simulink model "generic_IVS"  (R2024a)
settings: Solver=FixedStepDiscrete  StartTime=0.0  StopTime=inf  FixedStep=0.001  RelTol=1e-3  EnableMultiTasking=on
undefined symbols (not defined in the file): carLengthObs, dir, ego_Accel, ego_Speed, ego_X, ego_Y, ego_YAW, goalPosTol, goalYawTol, init_CurrentLaneInfo, init_DrivingMissionInfo, init_EgoVehicle, init_HybridAStarParam, init_MapData, init_ParkingMIssionInfo, is_Optimal_Path, isPathFound, LAD, lane_Coeff, lane_Idx, lane_waypoints, lane_waypoints_Length, lookAheadDistance, maxIter, missionState, obsRadius, parking_clear, parkingDestinationPos_X, parkingDestinationPos_Y, parkingDestinationYaw, parkingMapBoundary_X_Max, parkingMapBoundary_X_Min, parkingMapBoundary_Y_Max, parkingMapBoundary_Y_Min, parkingStartPos_X, parkingStartPos_Y, R_min, reversePenalty, Route1, route1_waypoint, Route2, route2_waypoint, Route3, route3_waypoint, Route_Parking, route_parking_waypoint, steerSet, stepSize, tollgateLaneNumber, vehicleRadius, velReference, xyResolution, y_LAD, y_lookAheadDistance, yawResolution, yawWeight
libraries: CarMaker4SL x53, simulink x1
(part 3 of 4)

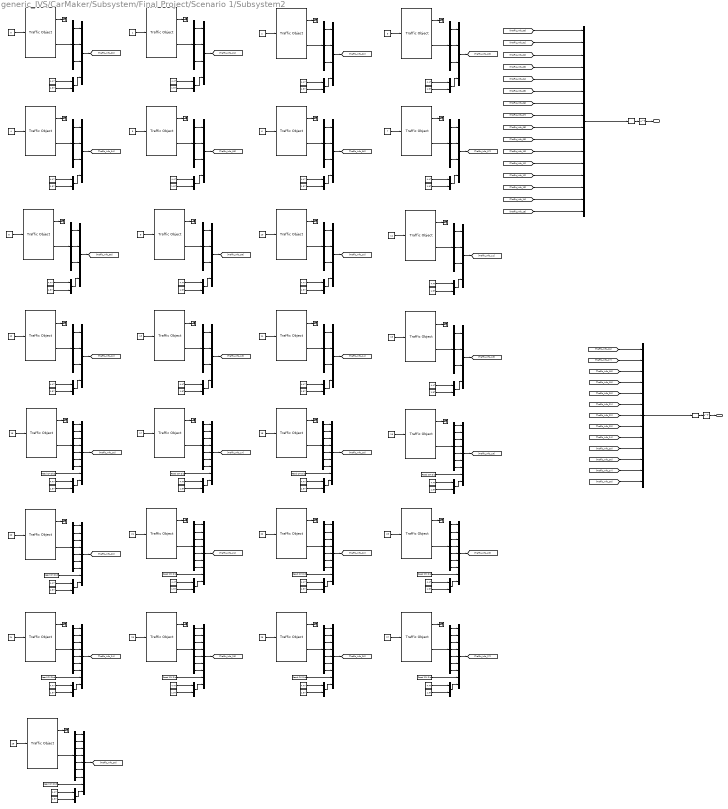
== system generic_IVS/CarMaker/Subsystem/Final Project/Scenario 1/Subsystem2 ==
  note: Traffic Size
      | Length: 4.47
      | Width: 1.97
      | Height: 1.12
  note: Traffic Size
      | Length: 4.47
      | Width: 1.97
      | Height: 1.12
  note: Traffic Size
      | Length: 4.47
      | Width: 1.97
      | Height: 1.12
  note: Traffic Size
      | Length: 4.47
      | Width: 1.97
      | Height: 1.12
  note: Traffic Size
      | Length: 4.47
      | Width: 1.97
      | Height: 1.12
  note: Traffic Size
      | Length: 4.47
      | Width: 1.97
      | Height: 1.12
  note: Traffic Size
      | Length: 4.47
      | Width: 1.97
      | Height: 1.12
  note: Traffic Size
      | Length: 4.47
      | Width: 1.97
      | Height: 1.12
  note: Traffic Size
      | Length: 4.47
      | Width: 1.97
      | Height: 1.12
  note: Traffic Size
      | Length: 4.47
      | Width: 1.97
      | Height: 1.12
  note: Traffic Size
      | Length: 4.47
      | Width: 1.97
      | Height: 1.12
  note: Traffic Size
      | Length: 4.47
      | Width: 1.97
      | Height: 1.12
  note: Traffic Size
      | Length: 4.47
      | Width: 1.97
      | Height: 1.12
  note: Traffic Size
      | Length: 4.47
      | Width: 1.97
      | Height: 1.12
  note: Traffic Size
      | Length: 4.47
      | Width: 1.97
      | Height: 1.12
  note: Traffic Size
      | Length: 4.47
      | Width: 1.97
      | Height: 1.12
  note: Traffic Size
      | Length: 4.47
      | Width: 1.97
      | Height: 1.12
  note: Traffic Size
      | Length: 4.47
      | Width: 1.97
      | Height: 1.12
  note: Traffic Size
      | Length: 4.47
      | Width: 1.97
      | Height: 1.12
  note: Traffic Size
      | Length: 4.47
      | Width: 1.97
      | Height: 1.12
  note: Traffic Size
      | Length: 4.47
      | Width: 1.97
      | Height: 1.12
  note: Traffic Size
      | Length: 4.47
      | Width: 1.97
      | Height: 1.12
  note: Traffic Size
      | Length: 4.47
      | Width: 1.97
      | Height: 1.12
  note: Traffic Size
      | Length: 4.47
      | Width: 1.97
      | Height: 1.12
  note: Traffic Size
      | Length: 4.47
      | Width: 1.97
      | Height: 1.12
  note: Traffic Size
      | Length: 4.47
      | Width: 1.97
      | Height: 1.12
  note: Traffic Size
      | Length: 4.47
      | Width: 1.97
      | Height: 1.12
  note: Traffic Size
      | Length: 4.47
      | Width: 1.97
      | Height: 1.12
  note: Traffic Size
      | Length: 4.47
      | Width: 1.97
      | Height: 1.12
  Bus Selector{1..14,19,29} (16 alike) : BusSelector  OutputSignals=t_0 x,t_0 y,r_zyx z
  Bus Selector{15..18,20..27,31} (13 alike) : BusSelector  OutputSignals=t_0 x,t_0 y,v_0 x,v_0 y,a_0 x,a_0 y,r_zyx z
  Constant1 : Constant
  Constant10 : Constant  Value=5
  Constant{2,5,8,11,14,17,19,23,26,29,31,35,38,41,43,47,50,53,55,59,62,65,67,71,74,77,79,89,94} (29 alike) : Constant  Value=4.47
  Constant{3,6,9,12,15,20..21,24,27,32..33,36,39,44..45,48,51,56..57,60,63,68..69,72,75,80..81,90,96} (29 alike) : Constant  Value=1.97
  Constant13 : Constant  Value=7
  Constant16 : Constant  Value=8
  Constant18 : Constant  Value=4
  Constant22 : Constant  Value=10
  Constant25 : Constant  Value=11
  Constant28 : Constant  Value=12
  Constant30 : Constant  Value=9
  Constant34 : Constant  Value=14
  Constant37 : Constant  Value=15
  Constant4 : Constant  Value=2
  Constant40 : Constant  Value=16
  Constant42 : Constant  Value=13
  Constant46 : Constant  Value=18
  Constant49 : Constant  Value=19
  Constant52 : Constant  Value=6
  Constant54 : Constant  Value=17
  Constant58 : Constant  Value=21
  Constant61 : Constant  Value=22
  Constant64 : Constant  Value=23
  Constant66 : Constant  Value=20
  Constant7 : Constant  Value=3
  Constant70 : Constant  Value=25
  Constant73 : Constant  Value=26
  Constant76 : Constant  Value=27
  Constant78 : Constant  Value=24
  Constant88 : Constant  Value=0
  Constant93 : Constant  Value=28
  Mux{1,3,5,7,10,12,14,16,18,20,22,24,26,30,36,60} (16 alike) : Mux
  Mux{2,4,6,8,11,13,15,17,19,21,23,25,27,29,31,33,35,37,39,41,43,45,47,49,51,53,55,61,65} (29 alike) : Mux  Inputs=2
  Mux{28,32,34,38,40,42,44,46,48,50,52,54,64} (13 alike) : Mux  Inputs=9
  Mux56 : Mux  Inputs=13
  Mux9 : Mux  Inputs=16
  Read CM Dict1 : CarMaker4SL/Read CM Dict  xname=Traffic.T20.rzv  xsync=off  xstime=Inherited
  Read CM Dict2 : CarMaker4SL/Read CM Dict  xname=Traffic.T18.rzv  xsync=off  xstime=Inherited
  Read CM Dict22 : CarMaker4SL/Read CM Dict  xname=Traffic.T21.rzv  xsync=off  xstime=Inherited
  Read CM Dict23 : CarMaker4SL/Read CM Dict  xname=Traffic.T22.rzv  xsync=off  xstime=Inherited
  Read CM Dict24 : CarMaker4SL/Read CM Dict  xname=Traffic.T23.rzv  xsync=off  xstime=Inherited
  Read CM Dict25 : CarMaker4SL/Read CM Dict  xname=Traffic.T24.rzv  xsync=off  xstime=Inherited
  Read CM Dict26 : CarMaker4SL/Read CM Dict  xname=Traffic.T25.rzv  xsync=off  xstime=Inherited
  Read CM Dict27 : CarMaker4SL/Read CM Dict  xname=Traffic.T26.rzv  xsync=off  xstime=Inherited
  Read CM Dict28 : CarMaker4SL/Read CM Dict  xname=Traffic.T27.rzv  xsync=off  xstime=Inherited
  Read CM Dict29 : CarMaker4SL/Read CM Dict  xname=Traffic.T28.rzv  xsync=off  xstime=Inherited
  Read CM Dict3 : CarMaker4SL/Read CM Dict  xname=Traffic.T17.rzv  xsync=off  xstime=Inherited
  Read CM Dict4 : CarMaker4SL/Read CM Dict  xname=Traffic.T16.rzv  xsync=off  xstime=Inherited
  Read CM Dict5 : CarMaker4SL/Read CM Dict  xname=Traffic.T19.rzv  xsync=off  xstime=Inherited
  Reshape : Reshape  OutputDimensionality=Customize  OutputDimensions=[5,16]
  Reshape1 : Reshape  OutputDimensionality=Customize  OutputDimensions=[10,13]
  Terminator{,1..28} (29 alike) : Terminator
  Traffic Object : CarMaker4SL/Traffic Object  xname=T00  ximode=Traffic Id  xstime=Inherited
      settings: SourceProductName=CarMaker4SL
  Traffic Object1 : CarMaker4SL/Traffic Object  xname=T01  ximode=Traffic Id  xstime=Inherited
      settings: SourceProductName=CarMaker4SL
  Traffic Object10 : CarMaker4SL/Traffic Object  xname=T11  ximode=Traffic Id  xstime=Inherited
      settings: SourceProductName=CarMaker4SL
  Traffic Object11 : CarMaker4SL/Traffic Object  xname=T12  ximode=Traffic Id  xstime=Inherited
      settings: SourceProductName=CarMaker4SL
  Traffic Object12 : CarMaker4SL/Traffic Object  xname=T13  ximode=Traffic Id  xstime=Inherited
      settings: SourceProductName=CarMaker4SL
  Traffic Object13 : CarMaker4SL/Traffic Object  xname=T14  ximode=Traffic Id  xstime=Inherited
      settings: SourceProductName=CarMaker4SL
  Traffic Object14 : CarMaker4SL/Traffic Object  xname=T15  ximode=Traffic Id  xstime=Inherited
      settings: SourceProductName=CarMaker4SL
  Traffic Object15 : CarMaker4SL/Traffic Object  xname=T16  ximode=Traffic Id  xstime=Inherited
      settings: SourceProductName=CarMaker4SL
  Traffic Object16 : CarMaker4SL/Traffic Object  xname=T17  ximode=Traffic Id  xstime=Inherited
      settings: SourceProductName=CarMaker4SL
  Traffic Object17 : CarMaker4SL/Traffic Object  xname=T18  ximode=Traffic Id  xstime=Inherited
      settings: SourceProductName=CarMaker4SL
  Traffic Object18 : CarMaker4SL/Traffic Object  xname=T19  ximode=Traffic Id  xstime=Inherited
      settings: SourceProductName=CarMaker4SL
  Traffic Object19 : CarMaker4SL/Traffic Object  xname=T06  ximode=Traffic Id  xstime=Inherited
      settings: SourceProductName=CarMaker4SL
  Traffic Object2 : CarMaker4SL/Traffic Object  xname=T02  ximode=Traffic Id  xstime=Inherited
      settings: SourceProductName=CarMaker4SL
  Traffic Object20 : CarMaker4SL/Traffic Object  xname=T20  ximode=Traffic Id  xstime=Inherited
      settings: SourceProductName=CarMaker4SL
  Traffic Object21 : CarMaker4SL/Traffic Object  xname=T21  ximode=Traffic Id  xstime=Inherited
      settings: SourceProductName=CarMaker4SL
  Traffic Object22 : CarMaker4SL/Traffic Object  xname=T22  ximode=Traffic Id  xstime=Inherited
      settings: SourceProductName=CarMaker4SL
  Traffic Object23 : CarMaker4SL/Traffic Object  xname=T23  ximode=Traffic Id  xstime=Inherited
      settings: SourceProductName=CarMaker4SL
  Traffic Object24 : CarMaker4SL/Traffic Object  xname=T24  ximode=Traffic Id  xstime=Inherited
      settings: SourceProductName=CarMaker4SL
  Traffic Object25 : CarMaker4SL/Traffic Object  xname=T25  ximode=Traffic Id  xstime=Inherited
      settings: SourceProductName=CarMaker4SL
  Traffic Object26 : CarMaker4SL/Traffic Object  xname=T26  ximode=Traffic Id  xstime=Inherited
      settings: SourceProductName=CarMaker4SL
  Traffic Object27 : CarMaker4SL/Traffic Object  xname=T27  ximode=Traffic Id  xstime=Inherited
      settings: SourceProductName=CarMaker4SL
  Traffic Object28 : CarMaker4SL/Traffic Object  xname=T28  ximode=Traffic Id  xstime=Inherited
      settings: SourceProductName=CarMaker4SL
  Traffic Object3 : CarMaker4SL/Traffic Object  xname=T03  ximode=Traffic Id  xstime=Inherited
      settings: SourceProductName=CarMaker4SL
  Traffic Object4 : CarMaker4SL/Traffic Object  xname=T04  ximode=Traffic Id  xstime=Inherited
      settings: SourceProductName=CarMaker4SL
  Traffic Object5 : CarMaker4SL/Traffic Object  xname=T05  ximode=Traffic Id  xstime=Inherited
      settings: SourceProductName=CarMaker4SL
  Traffic Object6 : CarMaker4SL/Traffic Object  xname=T07  ximode=Traffic Id  xstime=Inherited
      settings: SourceProductName=CarMaker4SL
  Traffic Object7 : CarMaker4SL/Traffic Object  xname=T08  ximode=Traffic Id  xstime=Inherited
      settings: SourceProductName=CarMaker4SL
  Traffic Object8 : CarMaker4SL/Traffic Object  xname=T09  ximode=Traffic Id  xstime=Inherited
      settings: SourceProductName=CarMaker4SL
  Traffic Object9 : CarMaker4SL/Traffic Object  xname=T10  ximode=Traffic Id  xstime=Inherited
      settings: SourceProductName=CarMaker4SL
  Transpose : Math  Operator=transpose
  Transpose1 : Math  Operator=transpose
  Traffic_Parking : Outport
  Traaffic_Info : Outport  Port=2
  wires:
  [Traffic_Info_00] -> Mux9/1
  [Traffic_Info_01] -> Mux9/2
  [Traffic_Info_02] -> Mux9/3
  [Traffic_Info_06] -> Mux9/7
  [Traffic_Info_05] -> Mux9/6
  [Traffic_Info_04] -> Mux9/5
  [Traffic_Info_03] -> Mux9/4
  [Traffic_Info_09] -> Mux9/10
  [Traffic_Info_10] -> Mux9/11
  [Traffic_Info_11] -> Mux9/12
  [Traffic_Info_08] -> Mux9/9
  [Traffic_Info_12] -> Mux9/13
  [Traffic_Info_13] -> Mux9/14
  [Traffic_Info_07] -> Mux9/8
  [Traffic_Info_15] -> Mux9/16
  [Traffic_Info_14] -> Mux9/15
  Traffic Object/2 -> Bus Selector29/1
  Constant88/1 -> Traffic Object/1
  Traffic Object/1 -> Terminator/1
  Bus Selector29/1 -> Mux60/1  "<t_0 x>"
  Bus Selector29/2 -> Mux60/2  "<t_0 y>"
  Bus Selector29/3 -> Mux60/3  "<r_zyx z>"
  Mux60/1 -> [Traffic_Info_00]
  Constant89/1 -> Mux61/1
  Constant90/1 -> Mux61/2
  Mux61/1 -> Mux60/4
  Bus Selector23/5 -> Mux44/5  "<a_0 x>"
  Traffic Object22/2 -> Bus Selector21/1
  Mux41/1 -> Mux40/9
  Constant63/1 -> Mux43/2
  Bus Selector23/2 -> Mux44/2  "<t_0 y>"
  Bus Selector21/2 -> Mux42/2  "<t_0 y>"
  Bus Selector21/5 -> Mux42/5  "<a_0 x>"
  Traffic Object22/1 -> Terminator22/1
  Bus Selector23/6 -> Mux44/6  "<a_0 y>"
  Bus Selector23/7 -> Mux44/7  "<r_zyx z>"
  Traffic Object23/1 -> Terminator23/1
  Traffic Object23/2 -> Bus Selector23/1
  Constant68/1 -> Mux45/2
  Mux45/1 -> Mux44/9
  Constant61/1 -> Traffic Object22/1
  Read CM Dict24/1 -> Mux44/8
  Mux42/1 -> [Traffic_Info_22]
  Mux40/1 -> [Traffic_Info_21]
  Mux44/1 -> [Traffic_Info_23]
  Bus Selector23/4 -> Mux44/4  "<v_0 y>"
  Bus Selector21/6 -> Mux42/6  "<a_0 y>"
  Bus Selector20/6 -> Mux40/6  "<a_0 y>"
  Bus Selector21/3 -> Mux42/3  "<v_0 x>"
  Bus Selector21/4 -> Mux42/4  "<v_0 y>"
  Bus Selector21/1 -> Mux42/1  "<t_0 x>"
  Constant58/1 -> Traffic Object21/1
  Bus Selector21/7 -> Mux42/7  "<r_zyx z>"
  Constant65/1 -> Mux45/1
  Bus Selector20/1 -> Mux40/1  "<t_0 x>"
  Bus Selector23/1 -> Mux44/1  "<t_0 x>"
  Bus Selector20/3 -> Mux40/3  "<v_0 x>"
  Constant60/1 -> Mux41/2
  Traffic Object21/2 -> Bus Selector20/1
  Read CM Dict22/1 -> Mux40/8
  Bus Selector20/5 -> Mux40/5  "<a_0 x>"
  Traffic Object21/1 -> Terminator21/1
  Bus Selector20/2 -> Mux40/2  "<t_0 y>"
  Bus Selector23/3 -> Mux44/3  "<v_0 x>"
  Constant64/1 -> Traffic Object23/1
  Bus Selector20/7 -> Mux40/7  "<r_zyx z>"
  Read CM Dict23/1 -> Mux42/8
  Constant62/1 -> Mux43/1
  Bus Selector20/4 -> Mux40/4  "<v_0 y>"
  Constant59/1 -> Mux41/1
  Mux43/1 -> Mux42/9
  Bus Selector26/3 -> Mux54/3  "<v_0 x>"
  Bus Selector27/5 -> Mux52/5  "<a_0 x>"
  Bus Selector26/5 -> Mux54/5  "<a_0 x>"
  Traffic Object26/2 -> Bus Selector25/1
  Bus Selector26/6 -> Mux54/6  "<a_0 y>"
  Mux49/1 -> Mux48/9
  Constant75/1 -> Mux51/2
  Bus Selector27/2 -> Mux52/2  "<t_0 y>"
  Bus Selector25/2 -> Mux50/2  "<t_0 y>"
  Bus Selector25/5 -> Mux50/5  "<a_0 x>"
  Traffic Object26/1 -> Terminator26/1
  Bus Selector27/6 -> Mux52/6  "<a_0 y>"
  Bus Selector26/7 -> Mux54/7  "<r_zyx z>"
  Bus Selector27/7 -> Mux52/7  "<r_zyx z>"
  Bus Selector26/1 -> Mux54/1  "<t_0 x>"
  Traffic Object27/1 -> Terminator27/1
  Traffic Object27/2 -> Bus Selector27/1
  Constant80/1 -> Mux53/2
  Mux53/1 -> Mux52/9
  Constant73/1 -> Traffic Object26/1
  Read CM Dict28/1 -> Mux52/8
  Mux50/1 -> [Traffic_Info_26]
  Mux48/1 -> [Traffic_Info_25]
  Mux52/1 -> [Traffic_Info_27]
  Bus Selector27/4 -> Mux52/4  "<v_0 y>"
  Constant78/1 -> Traffic Object24/1
  Traffic Object24/1 -> Terminator24/1
  Bus Selector25/6 -> Mux50/6  "<a_0 y>"
  Bus Selector24/6 -> Mux48/6  "<a_0 y>"
  Bus Selector25/3 -> Mux50/3  "<v_0 x>"
  Read CM Dict25/1 -> Mux54/8
  Bus Selector25/4 -> Mux50/4  "<v_0 y>"
  Bus Selector26/4 -> Mux54/4  "<v_0 y>"
  Bus Selector25/1 -> Mux50/1  "<t_0 x>"
  Constant70/1 -> Traffic Object25/1
  Bus Selector25/7 -> Mux50/7  "<r_zyx z>"
  Constant77/1 -> Mux53/1
  Bus Selector26/2 -> Mux54/2  "<t_0 y>"
  Bus Selector24/1 -> Mux48/1  "<t_0 x>"
  Bus Selector27/1 -> Mux52/1  "<t_0 x>"
  Bus Selector24/3 -> Mux48/3  "<v_0 x>"
  Mux54/1 -> [Traffic_Info_24]
  Constant72/1 -> Mux49/2
  Traffic Object25/2 -> Bus Selector24/1
  Read CM Dict26/1 -> Mux48/8
  Bus Selector24/5 -> Mux48/5  "<a_0 x>"
  Traffic Object25/1 -> Terminator25/1
  Constant81/1 -> Mux55/2
  Bus Selector24/2 -> Mux48/2  "<t_0 y>"
  Bus Selector27/3 -> Mux52/3  "<v_0 x>"
  Constant76/1 -> Traffic Object27/1
  Bus Selector24/7 -> Mux48/7  "<r_zyx z>"
  Traffic Object24/2 -> Bus Selector26/1
  Read CM Dict27/1 -> Mux50/8
  Mux55/1 -> Mux54/9
  Constant74/1 -> Mux51/1
  Bus Selector24/4 -> Mux48/4  "<v_0 y>"
  Constant71/1 -> Mux49/1
  Constant79/1 -> Mux55/1
  Mux51/1 -> Mux50/9
  Bus Selector31/3 -> Mux64/3  "<v_0 x>"
  Bus Selector31/5 -> Mux64/5  "<a_0 x>"
  Bus Selector31/6 -> Mux64/6  "<a_0 y>"
  Bus Selector31/7 -> Mux64/7  "<r_zyx z>"
  Bus Selector31/1 -> Mux64/1  "<t_0 x>"
  Constant93/1 -> Traffic Object28/1
  Traffic Object28/1 -> Terminator28/1
  Read CM Dict29/1 -> Mux64/8
  Bus Selector31/4 -> Mux64/4  "<v_0 y>"
  Bus Selector31/2 -> Mux64/2  "<t_0 y>"
  Mux64/1 -> [Traffic_Info_28]
  Constant96/1 -> Mux65/2
  Traffic Object28/2 -> Bus Selector31/1
  Mux65/1 -> Mux64/9
  Constant94/1 -> Mux65/1
  Bus Selector1/3 -> Mux1/3  "<r_zyx z>"
  Mux1/1 -> [Traffic_Info_01]
  Bus Selector1/1 -> Mux1/1  "<t_0 x>"
  Traffic Object1/1 -> Terminator1/1
  Constant2/1 -> Mux2/1
  Constant3/1 -> Mux2/2
  Bus Selector1/2 -> Mux1/2  "<t_0 y>"
  Mux2/1 -> Mux1/4
  Constant1/1 -> Traffic Object1/1
  Traffic Object1/2 -> Bus Selector1/1
  Bus Selector2/3 -> Mux3/3  "<r_zyx z>"
  Mux3/1 -> [Traffic_Info_02]
  Bus Selector2/1 -> Mux3/1  "<t_0 x>"
  Traffic Object2/1 -> Terminator2/1
  Constant5/1 -> Mux4/1
  Constant6/1 -> Mux4/2
  Bus Selector2/2 -> Mux3/2  "<t_0 y>"
  Mux4/1 -> Mux3/4
  Constant4/1 -> Traffic Object2/1
  Traffic Object2/2 -> Bus Selector2/1
  Bus Selector3/3 -> Mux5/3  "<r_zyx z>"
  Mux5/1 -> [Traffic_Info_03]
  Bus Selector3/1 -> Mux5/1  "<t_0 x>"
  Traffic Object3/1 -> Terminator3/1
  Constant8/1 -> Mux6/1
  Constant9/1 -> Mux6/2
  Bus Selector3/2 -> Mux5/2  "<t_0 y>"
  Mux6/1 -> Mux5/4
  Constant7/1 -> Traffic Object3/1
  Traffic Object3/2 -> Bus Selector3/1
  Bus Selector6/3 -> Mux14/3  "<r_zyx z>"
  Mux14/1 -> [Traffic_Info_04]
  Bus Selector6/1 -> Mux14/1  "<t_0 x>"
  Mux8/1 -> Mux7/4
  Constant12/1 -> Mux8/2
  Mux7/1 -> [Traffic_Info_05]
  Traffic Object4/1 -> Terminator4/1
  Bus Selector4/2 -> Mux7/2  "<t_0 y>"
  Constant18/1 -> Traffic Object4/1
  Constant21/1 -> Mux15/2
  Constant10/1 -> Traffic Object5/1
  Bus Selector6/2 -> Mux14/2  "<t_0 y>"
  Mux15/1 -> Mux14/4
  Traffic Object4/2 -> Bus Selector6/1
  Constant16/1 -> Traffic Object7/1
  Traffic Object7/2 -> Bus Selector7/1
  Constant17/1 -> Mux13/1
  Constant19/1 -> Mux15/1
  Constant11/1 -> Mux8/1
  Traffic Object7/1 -> Terminator7/1
  Constant20/1 -> Mux13/2
  Bus Selector4/1 -> Mux7/1  "<t_0 x>"
  Mux13/1 -> Mux12/4
  Bus Selector7/1 -> Mux12/1  "<t_0 x>"
  Bus Selector4/3 -> Mux7/3  "<r_zyx z>"
  Bus Selector7/3 -> Mux12/3  "<r_zyx z>"
  Mux12/1 -> [Traffic_Info_08]
  Constant15/1 -> Mux11/2
  Mux11/1 -> Mux10/4
  Constant13/1 -> Traffic Object6/1
  Traffic Object5/1 -> Terminator5/1
  Constant14/1 -> Mux11/1
  Traffic Object6/1 -> Terminator6/1
  Traffic Object5/2 -> Bus Selector4/1
  Bus Selector5/1 -> Mux10/1  "<t_0 x>"
  Bus Selector7/2 -> Mux12/2  "<t_0 y>"
  Traffic Object6/2 -> Bus Selector5/1
  Bus Selector5/3 -> Mux10/3  "<r_zyx z>"
  Mux10/1 -> [Traffic_Info_07]
  Bus Selector5/2 -> Mux10/2  "<t_0 y>"
  Bus Selector10/3 -> Mux22/3  "<r_zyx z>"
  Mux22/1 -> [Traffic_Info_09]
  Bus Selector10/1 -> Mux22/1  "<t_0 x>"
  Mux17/1 -> Mux16/4
  Constant24/1 -> Mux17/2
  Mux16/1 -> [Traffic_Info_10]
  Traffic Object8/1 -> Terminator8/1
  Bus Selector8/2 -> Mux16/2  "<t_0 y>"
  Constant30/1 -> Traffic Object8/1
  Constant33/1 -> Mux23/2
  Constant22/1 -> Traffic Object9/1
  Bus Selector10/2 -> Mux22/2  "<t_0 y>"
  Mux23/1 -> Mux22/4
  Traffic Object8/2 -> Bus Selector10/1
  Constant28/1 -> Traffic Object11/1
  Traffic Object11/2 -> Bus Selector11/1
  Constant29/1 -> Mux21/1
  Constant31/1 -> Mux23/1
  Constant23/1 -> Mux17/1
  Traffic Object11/1 -> Terminator11/1
  Constant32/1 -> Mux21/2
  Bus Selector8/1 -> Mux16/1  "<t_0 x>"
  Mux21/1 -> Mux20/4
  Bus Selector11/1 -> Mux20/1  "<t_0 x>"
  Bus Selector8/3 -> Mux16/3  "<r_zyx z>"
  Bus Selector11/3 -> Mux20/3  "<r_zyx z>"
  Mux20/1 -> [Traffic_Info_12]
  Constant27/1 -> Mux19/2
  Mux19/1 -> Mux18/4
  Constant25/1 -> Traffic Object10/1
  Traffic Object9/1 -> Terminator9/1
  Constant26/1 -> Mux19/1
  Traffic Object10/1 -> Terminator10/1
  Traffic Object9/2 -> Bus Selector8/1
  Bus Selector9/1 -> Mux18/1  "<t_0 x>"
  Bus Selector11/2 -> Mux20/2  "<t_0 y>"
  Traffic Object10/2 -> Bus Selector9/1
  Bus Selector9/3 -> Mux18/3  "<r_zyx z>"
  Mux18/1 -> [Traffic_Info_11]
  Bus Selector9/2 -> Mux18/2  "<t_0 y>"
  Bus Selector14/3 -> Mux30/3  "<r_zyx z>"
  Mux30/1 -> [Traffic_Info_13]
  Bus Selector14/1 -> Mux30/1  "<t_0 x>"
  Mux25/1 -> Mux24/4
  Constant36/1 -> Mux25/2
  Mux24/1 -> [Traffic_Info_14]
  Traffic Object12/1 -> Terminator12/1
  Bus Selector12/2 -> Mux24/2  "<t_0 y>"
  Constant42/1 -> Traffic Object12/1
  Constant45/1 -> Mux31/2
  Constant34/1 -> Traffic Object13/1
  Bus Selector14/2 -> Mux30/2  "<t_0 y>"
  Mux31/1 -> Mux30/4
  Traffic Object12/2 -> Bus Selector14/1
  Constant40/1 -> Traffic Object15/1
  Constant41/1 -> Mux29/1
  Constant43/1 -> Mux31/1
  Constant35/1 -> Mux25/1
  Traffic Object15/1 -> Terminator15/1
  Constant44/1 -> Mux29/2
  Bus Selector12/1 -> Mux24/1  "<t_0 x>"
  Mux29/1 -> Mux28/9
  Bus Selector12/3 -> Mux24/3  "<r_zyx z>"
  Mux28/1 -> [Traffic_Info_16]
  Constant39/1 -> Mux27/2
  Mux27/1 -> Mux26/4
  Constant37/1 -> Traffic Object14/1
  Traffic Object13/1 -> Terminator13/1
  Constant38/1 -> Mux27/1
  Traffic Object14/1 -> Terminator14/1
  Traffic Object13/2 -> Bus Selector12/1
  Bus Selector13/1 -> Mux26/1  "<t_0 x>"
  Traffic Object14/2 -> Bus Selector13/1
  Bus Selector13/3 -> Mux26/3  "<r_zyx z>"
  Mux26/1 -> [Traffic_Info_15]
  Bus Selector13/2 -> Mux26/2  "<t_0 y>"
  Traffic Object18/1 -> Terminator18/1
  Constant49/1 -> Traffic Object18/1
  Traffic Object17/1 -> Terminator17/1
  Constant50/1 -> Mux35/1
  Constant51/1 -> Mux35/2
  Constant55/1 -> Mux39/1
  Constant47/1 -> Mux33/1
  Mux39/1 -> Mux38/9
  Constant46/1 -> Traffic Object17/1
  Mux32/1 -> [Traffic_Info_18]
  Constant54/1 -> Traffic Object16/1
  Traffic Object16/1 -> Terminator16/1
  Constant48/1 -> Mux33/2
  Mux33/1 -> Mux32/9
  Constant57/1 -> Mux39/2
  Mux38/1 -> [Traffic_Info_17]
  Bus Selector19/1 -> Mux36/1  "<t_0 x>"
  Traffic Object19/1 -> Terminator19/1
  Constant53/1 -> Mux37/1
  Bus Selector19/2 -> Mux36/2  "<t_0 y>"
  Mux36/1 -> [Traffic_Info_06]
  Bus Selector19/3 -> Mux36/3  "<r_zyx z>"
  Traffic Object19/2 -> Bus Selector19/1
  Mux37/1 -> Mux36/4
  Constant52/1 -> Traffic Object19/1
  Constant56/1 -> Mux37/2
  Constant69/1 -> Mux47/2
  Traffic Object20/2 -> Bus Selector22/1
  Constant67/1 -> Mux47/1
  Constant66/1 -> Traffic Object20/1
  Traffic Object20/1 -> Terminator20/1
  Reshape/1 -> Transpose/1
  Transpose/1 -> Traffic_Parking/1
  Reshape1/1 -> Transpose1/1
  Transpose1/1 -> Traaffic_Info/1
  Mux9/1 -> Reshape/1
  Mux56/1 -> Reshape1/1
  Read CM Dict1/1 -> Mux46/8
  Bus Selector22/4 -> Mux46/4  "<v_0 y>"
  Bus Selector22/5 -> Mux46/5  "<a_0 x>"
  Bus Selector22/7 -> Mux46/7  "<r_zyx z>"
  Bus Selector22/2 -> Mux46/2  "<t_0 y>"
  Bus Selector22/3 -> Mux46/3  "<v_0 x>"
  Bus Selector22/1 -> Mux46/1  "<t_0 x>"
  Bus Selector22/6 -> Mux46/6  "<a_0 y>"
  Mux46/1 -> [Traffic_Info_20]
  Mux47/1 -> Mux46/9
  Bus Selector17/6 -> Mux34/6  "<a_0 y>"
  Bus Selector17/4 -> Mux34/4  "<v_0 y>"
  Mux34/1 -> [Traffic_Info_19]
  Bus Selector17/5 -> Mux34/5  "<a_0 x>"
  Bus Selector17/7 -> Mux34/7  "<r_zyx z>"
  Bus Selector17/3 -> Mux34/3  "<v_0 x>"
  Traffic Object18/2 -> Bus Selector17/1
  Bus Selector17/2 -> Mux34/2  "<t_0 y>"
  Bus Selector17/1 -> Mux34/1  "<t_0 x>"
  Read CM Dict5/1 -> Mux34/8
  Mux35/1 -> Mux34/9
  Bus Selector16/4 -> Mux32/4  "<v_0 y>"
  Bus Selector16/7 -> Mux32/7  "<r_zyx z>"
  Read CM Dict2/1 -> Mux32/8
  Bus Selector16/6 -> Mux32/6  "<a_0 y>"
  Bus Selector16/2 -> Mux32/2  "<t_0 y>"
  Traffic Object17/2 -> Bus Selector16/1
  Bus Selector16/1 -> Mux32/1  "<t_0 x>"
  Bus Selector16/3 -> Mux32/3  "<v_0 x>"
  Bus Selector16/5 -> Mux32/5  "<a_0 x>"
  Bus Selector18/4 -> Mux38/4  "<v_0 y>"
  Bus Selector18/7 -> Mux38/7  "<r_zyx z>"
  Read CM Dict3/1 -> Mux38/8
  Bus Selector18/6 -> Mux38/6  "<a_0 y>"
  Bus Selector18/2 -> Mux38/2  "<t_0 y>"
  Traffic Object16/2 -> Bus Selector18/1
  Bus Selector18/1 -> Mux38/1  "<t_0 x>"
  Bus Selector18/3 -> Mux38/3  "<v_0 x>"
  Bus Selector18/5 -> Mux38/5  "<a_0 x>"
  Bus Selector15/4 -> Mux28/4  "<v_0 y>"
  Bus Selector15/7 -> Mux28/7  "<r_zyx z>"
  Read CM Dict4/1 -> Mux28/8
  Bus Selector15/6 -> Mux28/6  "<a_0 y>"
  Bus Selector15/2 -> Mux28/2  "<t_0 y>"
  Traffic Object15/2 -> Bus Selector15/1
  Bus Selector15/1 -> Mux28/1  "<t_0 x>"
  Bus Selector15/3 -> Mux28/3  "<v_0 x>"
  Bus Selector15/5 -> Mux28/5  "<a_0 x>"
  [Traffic_Info_16] -> Mux56/1
  [Traffic_Info_17] -> Mux56/2
  [Traffic_Info_18] -> Mux56/3
  [Traffic_Info_19] -> Mux56/4
  [Traffic_Info_20] -> Mux56/5
  [Traffic_Info_21] -> Mux56/6
  [Traffic_Info_22] -> Mux56/7
  [Traffic_Info_23] -> Mux56/8
  [Traffic_Info_24] -> Mux56/9
  [Traffic_Info_25] -> Mux56/10
  [Traffic_Info_26] -> Mux56/11
  [Traffic_Info_27] -> Mux56/12
  [Traffic_Info_28] -> Mux56/13

== system generic_IVS/CarMaker/Subsystem/Final Project/Scenario 1/Subsystem3 ==
  In1 : Inport
  In2 : Inport  Port=2
  In3 : Inport  Port=3
  Bus Assignment : BusAssignment  AssignedSignals=parkingStartPos_X,parkingStartPos_Y,parkingDestinationPos_X,parkingDestinationPos_Y,parkingDestinationYaw,parkingMapBoundary_X_Min,parkingMapBoundary_X_Max,parkingMapBoundary_Y_Min,parkingMapBoundary_Y_Max,parking_clear,LAD,y_LAD,dir,isPathFound
  Bus Selector : BusSelector  OutputSignals=signal1,signal2
  Bus Selector1 : BusSelector  OutputSignals=signal1,signal2,signal3
  Bus Selector2 : BusSelector  OutputSignals=signal1,signal2,signal3,signal4
  Constant : Constant  Value=init_ParkingMIssionInfo  OutDataTypeStr=Bus: busParkingMissionInfo
  Constant1 : Constant  Value=0  OutDataTypeStr=uint8
  Constant2 : Constant  Value=0.01  OutDataTypeStr=single
  Constant3 : Constant  Value=0  OutDataTypeStr=single
  Constant4 : Constant  OutDataTypeStr=int8
  Constant5 : Constant  Value=0  OutDataTypeStr=uint8
  Out1 : Outport
  wires:
  Bus Assignment/1 -> [parking_mission_info]
  Constant/1 -> Bus Assignment/1
  In1/1 -> [startPoint]
  In2/1 -> [MapBoundary]
  In3/1 -> [endPose]
  [startPoint] -> Bus Selector/1
  Bus Selector/1 -> Bus Assignment/2  "<signal1>"
  Bus Selector/2 -> Bus Assignment/3  "<signal2>"
  [endPose] -> Bus Selector1/1
  Bus Selector1/1 -> Bus Assignment/4  "<signal1>"
  Bus Selector1/2 -> Bus Assignment/5  "<signal2>"
  Bus Selector1/3 -> Bus Assignment/6  "<signal3>"
  [MapBoundary] -> Bus Selector2/1
  Bus Selector2/1 -> Bus Assignment/7  "<signal1>"
  Bus Selector2/2 -> Bus Assignment/8  "<signal2>"
  Bus Selector2/3 -> Bus Assignment/9  "<signal3>"
  Bus Selector2/4 -> Bus Assignment/10  "<signal4>"
  [parking_mission_info] -> Out1/1
  Constant1/1 -> Bus Assignment/11
  Constant2/1 -> Bus Assignment/12
  Constant3/1 -> Bus Assignment/13
  Constant4/1 -> Bus Assignment/14
  Constant5/1 -> Bus Assignment/15

== system generic_IVS/CarMaker/Subsystem/Final Project/Scenario 1/Subsystem4 ==
  In1 : Inport
  Bus Assignment : BusAssignment  AssignedSignals=Route1,Route2,Route3,Route_Parking
  Bus Selector : BusSelector  OutputSignals=signal1,signal2,signal3,signal4
  Constant : Constant  Value=init_MapData  OutDataTypeStr=Bus: busMapData
  Out1 : Outport
  wires:
  Bus Assignment/1 -> [MapData_Info]
  [MapData_Info] -> Out1/1
  Constant/1 -> Bus Assignment/1
  In1/1 -> Bus Selector/1
  Bus Selector/1 -> Bus Assignment/2  "<signal1>"
  Bus Selector/2 -> Bus Assignment/3  "<signal2>"
  Bus Selector/3 -> Bus Assignment/4  "<signal3>"
  Bus Selector/4 -> Bus Assignment/5  "<signal4>"

== system generic_IVS/CarMaker/Subsystem/Final Project/Scenario 1/Subsystem5 ==
  In1 : Inport
  Bus Assignment : BusAssignment  AssignedSignals=missionState,tollgateLaneNumber,velReference,is_Optimal_Path
  Bus Selector : BusSelector  OutputSignals=signal1,signal2,signal3
  Constant : Constant  Value=init_DrivingMissionInfo  OutDataTypeStr=Bus: busDrivingMissionInfo
  Constant1 : Constant  Value=0  OutDataTypeStr=uint8
  Out1 : Outport
  wires:
  Constant/1 -> Bus Assignment/1
  Bus Assignment/1 -> [currentLaneInfo]
  [currentLaneInfo] -> Out1/1
  In1/1 -> [driving_mission_info_init]
  [driving_mission_info_init] -> Bus Selector/1
  Bus Selector/1 -> Bus Assignment/2  "<signal1>"
  Bus Selector/2 -> Bus Assignment/3  "<signal2>"
  Bus Selector/3 -> Bus Assignment/4  "<signal3>"
  Constant1/1 -> Bus Assignment/5

== system generic_IVS/CarMaker/Subsystem/Final Project/Scenario 1/Subsystem6 ==
  note: 바운더리 앞에 있으면 1
      | 바운더리 뒤에 있으면 0
  In1 : Inport
  Bus Creator : BusCreator  Inputs=3
  Constant6 : Constant
  Constant7 : Constant  Value=0
  Display10 : Display
  Display4 : Display
  Display5 : Display
  MATLAB Function10 : MATLAB Function  TreatAsAtomicUnit=on
  MATLAB Function11 : MATLAB Function  TreatAsAtomicUnit=on
  MATLAB Function9 : MATLAB Function  TreatAsAtomicUnit=on
  Manual Switch1 : ManualSwitch
  Out1 : Outport
  wires:
  Constant6/1 -> Manual Switch1/1
  Manual Switch1/1 -> MATLAB Function10/2(IS_FRONT)
  MATLAB Function11/1(parking_mode) -> Display5/1, [state_4_flag]
  MATLAB Function9/1(tollgate_pass_mode) -> [state_2_flag], Display4/1
  [Ego_Status] -> MATLAB Function11/1(ego_status)
  MATLAB Function10/1(parking_entry_mode) -> Display10/1, [state_3_flag]
  [Ego_Status] -> MATLAB Function9/1(ego_status)
  Constant7/1 -> Manual Switch1/2
  [Ego_Status] -> MATLAB Function10/1(ego_status)
  In1/1 -> [Ego_Status]
  [state_2_flag] -> Bus Creator/1
  [state_3_flag] -> Bus Creator/2
  [state_4_flag] -> Bus Creator/3
  Bus Creator/1 -> [state_flag]
  [state_flag] -> Out1/1

== system generic_IVS/CarMaker/Subsystem/Final Project/Scenario 1/Subsystem7 ==
  In1 : Inport
  In2 : Inport  Port=2
  In3 : Inport  Port=3
  Bus Assignment : BusAssignment  AssignedSignals=missionState
  Bus Selector1 : BusSelector  OutputSignals=tollgate_pass_mode,parking_entry_mode,parking_mode
  Chart3 : Stateflow chart  TreatAsAtomicUnit=on
  Display9 : Display
  Switch : Switch  Criteria=u2 > Threshold  SaturateOnIntegerOverflow=off  InputSameDT=off
  Out1 : Outport
  wires:
  Bus Selector1/3 -> Chart3/3(flag_4)  "<parking_mode>"
  Chart3/1(mission) -> [state], Display9/1
  Bus Selector1/2 -> Chart3/2(flag_3)  "<parking_entry_mode>"
  Bus Selector1/1 -> Chart3/1(flag_2)  "<tollgate_pass_mode>"
  In1/1 -> Bus Selector1/1
  [driving_mission_info] -> Bus Assignment/1
  Bus Assignment/1 -> Out1/1
  In2/1 -> [driving_mission_info]
  In3/1 -> [missionState_forced]
  [missionState_forced] -> Switch/2
  [missionState_forced] -> Switch/1
  [state] -> Switch/3
  Switch/1 -> Bus Assignment/2

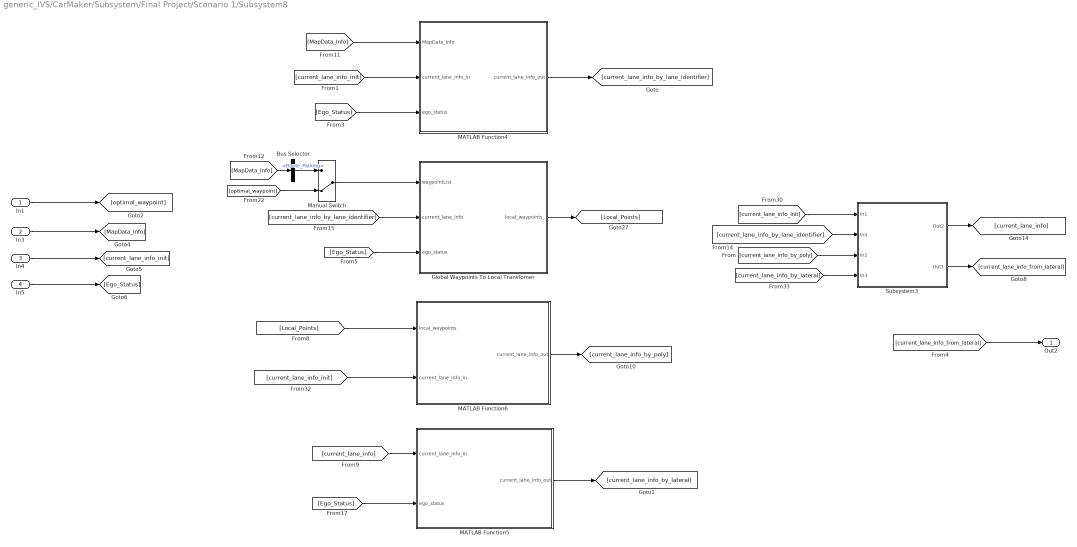
== system generic_IVS/CarMaker/Subsystem/Final Project/Scenario 1/Subsystem8 ==
  In1 : Inport
  In3 : Inport  Port=2
  In4 : Inport  Port=3
  In5 : Inport  Port=4
  Bus Selector : BusSelector  OutputSignals=Route_Parking
  Global Waypoints To Local Transfomer : MATLAB Function  TreatAsAtomicUnit=on
  MATLAB Function4 : MATLAB Function  TreatAsAtomicUnit=on
  MATLAB Function5 : MATLAB Function  TreatAsAtomicUnit=on
  MATLAB Function6 : MATLAB Function  TreatAsAtomicUnit=on
  Manual Switch : ManualSwitch  CurrentSetting=0  varsize=on
  Subsystem3 : Subsystem
  Out2 : Outport
  wires:
  [optimal_waypoint] -> Manual Switch/2
  [current_lane_info_by_lane_identifier] -> Global Waypoints To Local Transfomer/2(current_lane_info)
  Subsystem3/2(Out1) -> [current_lane_info_from_lateral]
  MATLAB Function5/1(current_lane_info_out) -> [current_lane_info_by_lateral]
  MATLAB Function6/1(current_lane_info_out) -> [current_lane_info_by_poly]
  [current_lane_info] -> MATLAB Function5/1(current_lane_info_in)
  MATLAB Function4/1(current_lane_info_out) -> [current_lane_info_by_lane_identifier]
  [Local_Points] -> MATLAB Function6/1(local_waypoints)
  [current_lane_info_by_lane_identifier] -> Subsystem3/2(In4)
  Subsystem3/1(Out2) -> [current_lane_info]
  [Ego_Status] -> MATLAB Function4/3(ego_status)
  Manual Switch/1 -> Global Waypoints To Local Transfomer/1(waypointList)
  [current_lane_info_init] -> MATLAB Function4/2(current_lane_info_in)
  [current_lane_info_by_poly] -> Subsystem3/3(In2)
  [current_lane_info_by_lateral] -> Subsystem3/4(In3)
  Global Waypoints To Local Transfomer/1(local_waypoints_) -> [Local_Points]
  [Ego_Status] -> Global Waypoints To Local Transfomer/3(ego_status)
  [MapData_Info] -> MATLAB Function4/1(MapData_Info)
  Bus Selector/1 -> Manual Switch/1  "<Route_Parking>"
  [MapData_Info] -> Bus Selector/1
  [current_lane_info_init] -> Subsystem3/1(In1)
  [current_lane_info_init] -> MATLAB Function6/2(current_lane_info_in)
  [Ego_Status] -> MATLAB Function5/2(ego_status)
  [current_lane_info_from_lateral] -> Out2/1
  In1/1 -> [optimal_waypoint]
  In3/1 -> [MapData_Info]
  In4/1 -> [current_lane_info_init]
  In5/1 -> [Ego_Status]

== system generic_IVS/CarMaker/Subsystem/Final Project/Scenario 1/Subsystem9 ==
  In1 : Inport  OutDataTypeStr=Bus: busCurrentLaneInfo
  In2 : Inport  Port=2
  In3 : Inport  Port=3
  Lateral Control : Subsystem
  Longiutidnal Control : Subsystem
  Out1 : Outport
  Out2 : Outport  Port=2
  wires:
  [Ego_Status] -> Lateral Control/2(In1)
  [current_lane_info_from_lateral] -> Lateral Control/1(In3)
  Lateral Control/1(Out1) -> [delta]
  [delta] -> Out2/1
  In1/1 -> [current_lane_info_from_lateral]
  In2/1 -> [Ego_Status]
  In3/1 -> [driving_mission_info_by_planner]
  Longiutidnal Control/1(1) -> [desired_ax]
  [Ego_Status] -> Longiutidnal Control/1(In2)
  [driving_mission_info_by_planner] -> Longiutidnal Control/2(In3)
  [desired_ax] -> Out1/1

== system generic_IVS/CarMaker/IPG Vehicle/CarAndTrailer/Forces/Suspension Forces/Suspension External Forces Update ==
  Bus Creator21 : BusCreator  Inputs=6
  Bus Creator22 : BusCreator  Inputs=4
  Bus Creator23 : BusCreator  Inputs=4
  From : From  TagVisibility=global
  Ground{32..39} (8 alike) : Ground
  Out1 : Outport
  wires:
  [D] -> Bus Creator21/4
  Ground36/1 -> Bus Creator22/1
  From/1 -> Bus Creator21/1
  [B] -> Bus Creator21/2
  Ground34/1 -> Bus Creator23/3
  Ground32/1 -> Bus Creator23/1
  [C] -> Bus Creator21/3
  Bus Creator23/1 -> Bus Creator21/5
  Ground33/1 -> Bus Creator23/2
  Bus Creator22/1 -> Bus Creator21/6
  Bus Creator21/1 -> Out1/1
  Ground35/1 -> Bus Creator23/4
  Ground39/1 -> Bus Creator22/4
  Ground38/1 -> Bus Creator22/3
  Ground37/1 -> Bus Creator22/2

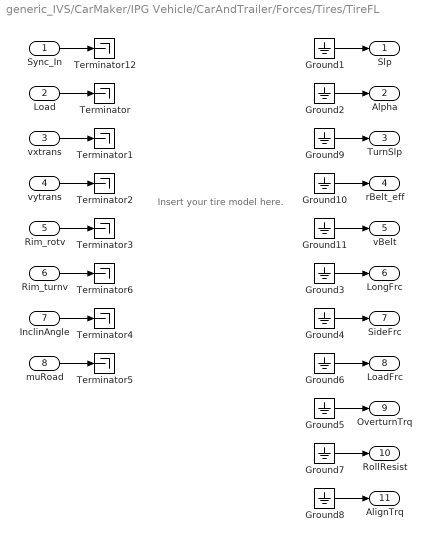
== system generic_IVS/CarMaker/IPG Vehicle/CarAndTrailer/Forces/Tires/TireFL ==
  note: Insert your tire model here.
  Sync_In : Inport
  Load : Inport  Port=2
  vxtrans : Inport  Port=3
  vytrans : Inport  Port=4
  Rim_rotv : Inport  Port=5
  Rim_turnv : Inport  Port=6
  InclinAngle : Inport  Port=7
  muRoad : Inport  Port=8
  Ground{1..11} (11 alike) : Ground
  Terminator{,1..6,12} (8 alike) : Terminator
  Slp : Outport  VectorParamsAs1DForOutWhenUnconnected=off
  Alpha : Outport  Port=2  VectorParamsAs1DForOutWhenUnconnected=off
  TurnSlp : Outport  Port=3  VectorParamsAs1DForOutWhenUnconnected=off
  rBelt_eff : Outport  Port=4  VectorParamsAs1DForOutWhenUnconnected=off
  vBelt : Outport  Port=5  VectorParamsAs1DForOutWhenUnconnected=off
  LongFrc : Outport  Port=6  VectorParamsAs1DForOutWhenUnconnected=off
  SideFrc : Outport  Port=7  VectorParamsAs1DForOutWhenUnconnected=off
  LoadFrc : Outport  Port=8  VectorParamsAs1DForOutWhenUnconnected=off
  OverturnTrq : Outport  Port=9  VectorParamsAs1DForOutWhenUnconnected=off
  RollResist : Outport  Port=10  VectorParamsAs1DForOutWhenUnconnected=off
  AlignTrq : Outport  Port=11  VectorParamsAs1DForOutWhenUnconnected=off
  wires:
  Ground11/1 -> vBelt/1
  Ground10/1 -> rBelt_eff/1
  Ground9/1 -> TurnSlp/1
  Rim_turnv/1 -> Terminator6/1
  Sync_In/1 -> Terminator12/1
  Ground2/1 -> Alpha/1
  Ground3/1 -> LongFrc/1
  Ground4/1 -> SideFrc/1
  Ground5/1 -> OverturnTrq/1
  vxtrans/1 -> Terminator1/1
  vytrans/1 -> Terminator2/1
  Rim_rotv/1 -> Terminator3/1
  InclinAngle/1 -> Terminator4/1
  muRoad/1 -> Terminator5/1
  Load/1 -> Terminator/1
  Ground1/1 -> Slp/1
  Ground6/1 -> LoadFrc/1
  Ground7/1 -> RollResist/1
  Ground8/1 -> AlignTrq/1

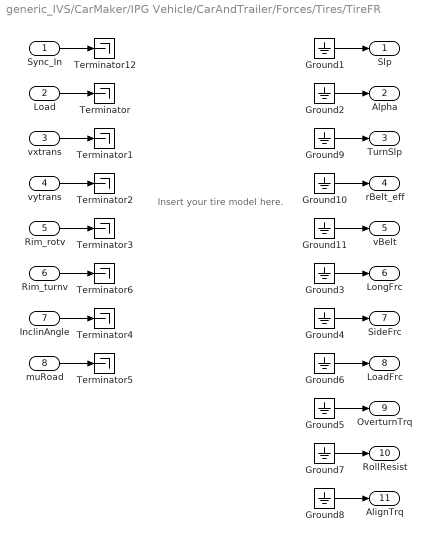
== system generic_IVS/CarMaker/IPG Vehicle/CarAndTrailer/Forces/Tires/TireFR ==
  note: Insert your tire model here.
  Sync_In : Inport
  Load : Inport  Port=2
  vxtrans : Inport  Port=3
  vytrans : Inport  Port=4
  Rim_rotv : Inport  Port=5
  Rim_turnv : Inport  Port=6
  InclinAngle : Inport  Port=7
  muRoad : Inport  Port=8
  Ground{1..11} (11 alike) : Ground
  Terminator{,1..6,12} (8 alike) : Terminator
  Slp : Outport  VectorParamsAs1DForOutWhenUnconnected=off
  Alpha : Outport  Port=2  VectorParamsAs1DForOutWhenUnconnected=off
  TurnSlp : Outport  Port=3  VectorParamsAs1DForOutWhenUnconnected=off
  rBelt_eff : Outport  Port=4  VectorParamsAs1DForOutWhenUnconnected=off
  vBelt : Outport  Port=5  VectorParamsAs1DForOutWhenUnconnected=off
  LongFrc : Outport  Port=6  VectorParamsAs1DForOutWhenUnconnected=off
  SideFrc : Outport  Port=7  VectorParamsAs1DForOutWhenUnconnected=off
  LoadFrc : Outport  Port=8  VectorParamsAs1DForOutWhenUnconnected=off
  OverturnTrq : Outport  Port=9  VectorParamsAs1DForOutWhenUnconnected=off
  RollResist : Outport  Port=10  VectorParamsAs1DForOutWhenUnconnected=off
  AlignTrq : Outport  Port=11  VectorParamsAs1DForOutWhenUnconnected=off
  wires:
  Ground11/1 -> vBelt/1
  Ground10/1 -> rBelt_eff/1
  Ground9/1 -> TurnSlp/1
  Rim_turnv/1 -> Terminator6/1
  Sync_In/1 -> Terminator12/1
  Ground2/1 -> Alpha/1
  Ground3/1 -> LongFrc/1
  Ground4/1 -> SideFrc/1
  Ground5/1 -> OverturnTrq/1
  vxtrans/1 -> Terminator1/1
  vytrans/1 -> Terminator2/1
  Rim_rotv/1 -> Terminator3/1
  InclinAngle/1 -> Terminator4/1
  muRoad/1 -> Terminator5/1
  Load/1 -> Terminator/1
  Ground1/1 -> Slp/1
  Ground6/1 -> LoadFrc/1
  Ground7/1 -> RollResist/1
  Ground8/1 -> AlignTrq/1

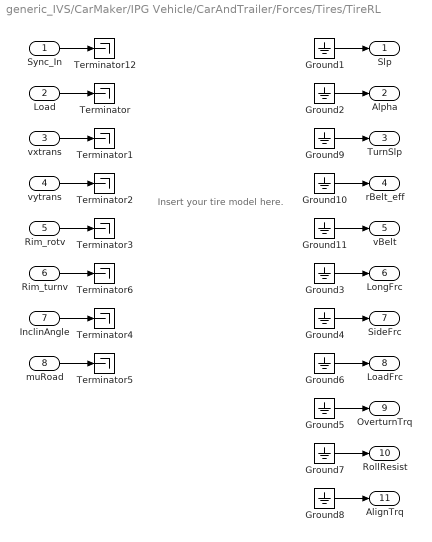
== system generic_IVS/CarMaker/IPG Vehicle/CarAndTrailer/Forces/Tires/TireRL ==
  note: Insert your tire model here.
  Sync_In : Inport
  Load : Inport  Port=2
  vxtrans : Inport  Port=3
  vytrans : Inport  Port=4
  Rim_rotv : Inport  Port=5
  Rim_turnv : Inport  Port=6
  InclinAngle : Inport  Port=7
  muRoad : Inport  Port=8
  Ground{1..11} (11 alike) : Ground
  Terminator{,1..6,12} (8 alike) : Terminator
  Slp : Outport  VectorParamsAs1DForOutWhenUnconnected=off
  Alpha : Outport  Port=2  VectorParamsAs1DForOutWhenUnconnected=off
  TurnSlp : Outport  Port=3  VectorParamsAs1DForOutWhenUnconnected=off
  rBelt_eff : Outport  Port=4  VectorParamsAs1DForOutWhenUnconnected=off
  vBelt : Outport  Port=5  VectorParamsAs1DForOutWhenUnconnected=off
  LongFrc : Outport  Port=6  VectorParamsAs1DForOutWhenUnconnected=off
  SideFrc : Outport  Port=7  VectorParamsAs1DForOutWhenUnconnected=off
  LoadFrc : Outport  Port=8  VectorParamsAs1DForOutWhenUnconnected=off
  OverturnTrq : Outport  Port=9  VectorParamsAs1DForOutWhenUnconnected=off
  RollResist : Outport  Port=10  VectorParamsAs1DForOutWhenUnconnected=off
  AlignTrq : Outport  Port=11  VectorParamsAs1DForOutWhenUnconnected=off
  wires:
  Ground11/1 -> vBelt/1
  Ground10/1 -> rBelt_eff/1
  Ground9/1 -> TurnSlp/1
  Rim_turnv/1 -> Terminator6/1
  Sync_In/1 -> Terminator12/1
  Ground2/1 -> Alpha/1
  Ground3/1 -> LongFrc/1
  Ground4/1 -> SideFrc/1
  Ground5/1 -> OverturnTrq/1
  vxtrans/1 -> Terminator1/1
  vytrans/1 -> Terminator2/1
  Rim_rotv/1 -> Terminator3/1
  InclinAngle/1 -> Terminator4/1
  muRoad/1 -> Terminator5/1
  Load/1 -> Terminator/1
  Ground1/1 -> Slp/1
  Ground6/1 -> LoadFrc/1
  Ground7/1 -> RollResist/1
  Ground8/1 -> AlignTrq/1

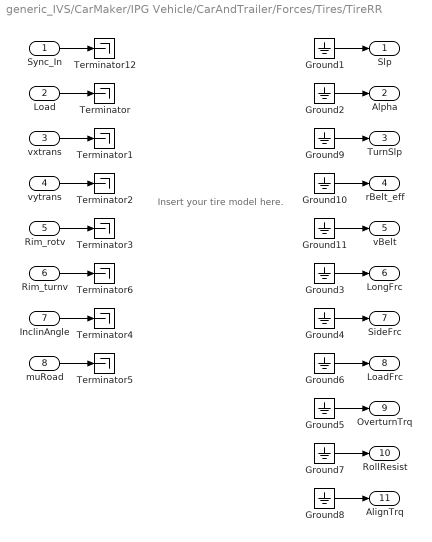
== system generic_IVS/CarMaker/IPG Vehicle/CarAndTrailer/Forces/Tires/TireRR ==
  note: Insert your tire model here.
  Sync_In : Inport
  Load : Inport  Port=2
  vxtrans : Inport  Port=3
  vytrans : Inport  Port=4
  Rim_rotv : Inport  Port=5
  Rim_turnv : Inport  Port=6
  InclinAngle : Inport  Port=7
  muRoad : Inport  Port=8
  Ground{1..11} (11 alike) : Ground
  Terminator{,1..6,12} (8 alike) : Terminator
  Slp : Outport  VectorParamsAs1DForOutWhenUnconnected=off
  Alpha : Outport  Port=2  VectorParamsAs1DForOutWhenUnconnected=off
  TurnSlp : Outport  Port=3  VectorParamsAs1DForOutWhenUnconnected=off
  rBelt_eff : Outport  Port=4  VectorParamsAs1DForOutWhenUnconnected=off
  vBelt : Outport  Port=5  VectorParamsAs1DForOutWhenUnconnected=off
  LongFrc : Outport  Port=6  VectorParamsAs1DForOutWhenUnconnected=off
  SideFrc : Outport  Port=7  VectorParamsAs1DForOutWhenUnconnected=off
  LoadFrc : Outport  Port=8  VectorParamsAs1DForOutWhenUnconnected=off
  OverturnTrq : Outport  Port=9  VectorParamsAs1DForOutWhenUnconnected=off
  RollResist : Outport  Port=10  VectorParamsAs1DForOutWhenUnconnected=off
  AlignTrq : Outport  Port=11  VectorParamsAs1DForOutWhenUnconnected=off
  wires:
  Ground11/1 -> vBelt/1
  Ground10/1 -> rBelt_eff/1
  Ground9/1 -> TurnSlp/1
  Rim_turnv/1 -> Terminator6/1
  Sync_In/1 -> Terminator12/1
  Ground2/1 -> Alpha/1
  Ground3/1 -> LongFrc/1
  Ground4/1 -> SideFrc/1
  Ground5/1 -> OverturnTrq/1
  vxtrans/1 -> Terminator1/1
  vytrans/1 -> Terminator2/1
  Rim_rotv/1 -> Terminator3/1
  InclinAngle/1 -> Terminator4/1
  muRoad/1 -> Terminator5/1
  Load/1 -> Terminator/1
  Ground1/1 -> Slp/1
  Ground6/1 -> LoadFrc/1
  Ground7/1 -> RollResist/1
  Ground8/1 -> AlignTrq/1

== system generic_IVS/CarMaker/Subsystem/Final Project/Scenario 1/Subsystem11/Lateral Control ==
  In3 : Inport  OutDataTypeStr=Bus: busParkingMissionInfo
  In1 : Inport  Port=2
  Data Type Conversion6 : DataTypeConversion  OutDataTypeStr=double  SaturateOnIntegerOverflow=off  RndMeth=Floor
  MATLAB Function8 : MATLAB Function  TreatAsAtomicUnit=on
  Saturation2 : Saturate  UpperLimit=1  LowerLimit=-1
  Out1 : Outport
  wires:
  [parking_mission_info] -> MATLAB Function8/1(parking_mission_info)
  MATLAB Function8/1(delta) -> Data Type Conversion6/1
  Data Type Conversion6/1 -> Saturation2/1
  Saturation2/1 -> Out1/1  "delta"
  In3/1 -> [parking_mission_info]
  In1/1 -> [Ego_Status]
  [Ego_Status] -> MATLAB Function8/2(ego_status)

== system generic_IVS/CarMaker/Subsystem/Final Project/Scenario 1/Subsystem11/Longiutidnal Control ==
  In2 : Inport
  In3 : Inport  Port=2
  Bus Selector : BusSelector  OutputSignals=dir,parking_clear
  Data Type Conversion1 : DataTypeConversion  OutDataTypeStr=double  SaturateOnIntegerOverflow=off  RndMeth=Floor
  Data Type Conversion2 : DataTypeConversion  OutDataTypeStr=double  SaturateOnIntegerOverflow=off  RndMeth=Floor
  Data Type Conversion5 : DataTypeConversion  OutDataTypeStr=double  SaturateOnIntegerOverflow=off  RndMeth=Floor
  Gain : Gain  Gain=1000
  Longitudinal PI Controller : MATLAB Function  TreatAsAtomicUnit=on
  Write CM Dict : CarMaker4SL/Write CM Dict  xname=DM.SelectorCtrl  xsync=off
  Write CM Dict1 : CarMaker4SL/Write CM Dict  xname=DM.Brake  xsync=off
  1 : Outport
  wires:
  Longitudinal PI Controller/1(desired_ax) -> Data Type Conversion5/1
  [parking_mission_info] -> Longitudinal PI Controller/2(parking_mission_info)
  [Ego_Status] -> Longitudinal PI Controller/1(ego_status)
  Data Type Conversion5/1 -> 1/1  "input a_x"
  In2/1 -> [Ego_Status]
  In3/1 -> [parking_mission_info]
  [parking_mission_info] -> Bus Selector/1
  Bus Selector/1 -> Data Type Conversion1/1  "<dir>"
  Data Type Conversion1/1 -> Write CM Dict/1
  Bus Selector/2 -> Data Type Conversion2/1  "<parking_clear>"
  Data Type Conversion2/1 -> Gain/1
  Gain/1 -> Write CM Dict1/1

== system generic_IVS/CarMaker/Subsystem/Final Project/Scenario 1/Subsystem8/Subsystem3 ==
  In1 : Inport  OutDataTypeStr=Bus: busCurrentLaneInfo
  In4 : Inport  Port=2  OutDataTypeStr=Bus: busCurrentLaneInfo
  In2 : Inport  Port=3  OutDataTypeStr=Bus: busCurrentLaneInfo
  In3 : Inport  Port=4  OutDataTypeStr=Bus: busCurrentLaneInfo
  Bus Assignment : BusAssignment  AssignedSignals=lane_Coeff,lane_Idx,lane_waypoints,lane_waypoints_Length
  Bus Assignment1 : BusAssignment  AssignedSignals=lookAheadDistance,y_lookAheadDistance
  Bus Creator : BusCreator  Inputs=2
  Bus Selector : BusSelector  OutputSignals=lookAheadDistance,y_lookAheadDistance
  Bus Selector1 : BusSelector  OutputSignals=by_poly.lane_Coeff,by_identifier.lane_Idx,by_identifier.lane_waypoints,by_identifier.lane_waypoints_Length
  Out2 : Outport  OutDataTypeStr=Bus: busCurrentLaneInfo
  Out1 : Outport  Port=2  OutDataTypeStr=Bus: busCurrentLaneInfo
  wires:
  [current_lane_info_init] -> Bus Assignment/1
  Bus Assignment/1 -> [current_lane_info], Bus Assignment1/1
  In1/1 -> [current_lane_info_init]
  Bus Assignment1/1 -> [current_lane_info_from_lateral]
  Bus Selector1/1 -> Bus Assignment/2  "<lane_Coeff>"
  In2/1 -> [current_lane_info_by_poly]
  [current_lane_info_by_lateral] -> Bus Selector/1
  In3/1 -> [current_lane_info_by_lateral]
  [current_lane_info] -> Out2/1
  [current_lane_info_from_lateral] -> Out1/1
  Bus Selector/1 -> Bus Assignment1/2  "<lookAheadDistance>"
  Bus Selector/2 -> Bus Assignment1/3  "<y_lookAheadDistance>"
  In4/1 -> [current_lane_info_by_lane_identifier]
  [current_lane_info_by_poly] -> Bus Creator/1  "by_poly"
  [current_lane_info_by_lane_identifier] -> Bus Creator/2  "by_identifier"
  Bus Creator/1 -> Bus Selector1/1
  Bus Selector1/2 -> Bus Assignment/3  "<lane_Idx>"
  Bus Selector1/3 -> Bus Assignment/4  "<lane_waypoints>"
  Bus Selector1/4 -> Bus Assignment/5  "<lane_waypoints_Length>"

== system generic_IVS/CarMaker/Subsystem/Final Project/Scenario 1/Subsystem9/Lateral Control ==
  In3 : Inport  OutDataTypeStr=Bus: busCurrentLaneInfo
  In1 : Inport  Port=2
  Data Type Conversion6 : DataTypeConversion  OutDataTypeStr=double  SaturateOnIntegerOverflow=off  RndMeth=Floor
  Data Type Conversion7 : DataTypeConversion  Commented=on  OutDataTypeStr=double  SaturateOnIntegerOverflow=off  RndMeth=Floor
  From25 : From  Commented=on  GotoTag=Ego_Status
  From26 : From  Commented=on  GotoTag=current_lane_info_from_lateral
  MATLAB Function7 : MATLAB Function  Commented=on  TreatAsAtomicUnit=on
  MATLAB Function8 : MATLAB Function  TreatAsAtomicUnit=on
  Saturation1 : Saturate  Commented=on  UpperLimit=35*180/pi  LowerLimit=-35*180/pi
  Saturation2 : Saturate  UpperLimit=1  LowerLimit=-1
  Out1 : Outport
  wires:
  [current_lane_info_from_lateral] -> MATLAB Function8/1(current_lane_info)
  MATLAB Function8/1(delta) -> Data Type Conversion6/1
  Data Type Conversion6/1 -> Saturation2/1
  From26/1 -> MATLAB Function7/1(current_lane_info)
  Saturation2/1 -> Out1/1  "delta"
  MATLAB Function7/1(delta) -> Data Type Conversion7/1
  From25/1 -> MATLAB Function7/2(ego_status)
  Saturation1/1 -> ?
  Data Type Conversion7/1 -> Saturation1/1
  In3/1 -> [current_lane_info_from_lateral]
  In1/1 -> [Ego_Status]

== system generic_IVS/CarMaker/Subsystem/Final Project/Scenario 1/Subsystem9/Longiutidnal Control ==
  In2 : Inport
  In3 : Inport  Port=2
  Data Type Conversion5 : DataTypeConversion  OutDataTypeStr=double  SaturateOnIntegerOverflow=off  RndMeth=Floor
  Longitudinal PI Controller : MATLAB Function  TreatAsAtomicUnit=on
  1 : Outport
  wires:
  Longitudinal PI Controller/1(desired_ax) -> Data Type Conversion5/1
  [driving_mission_info_by_planner] -> Longitudinal PI Controller/2(driving_mission_info)
  [Ego_Status] -> Longitudinal PI Controller/1(ego_status)
  Data Type Conversion5/1 -> 1/1  "input a_x"
  In2/1 -> [Ego_Status]
  In3/1 -> [driving_mission_info_by_planner]

== matlab function generic_IVS/CarMaker/Subsystem/Final Project/Scenario 1/Subsystem11/Longiutidnal Control/Longitudinal PI Controller ==
  settings: updateMethod=DISCRETE  sampleTime=0.01
  data: desired_ax output; ego_status input Bus: busEgoVehicle; parking_mission_info input Bus: busParkingMissionInfo
function desired_ax = longitudinal_speed_pi_controller_parking(ego_status, parking_mission_info)
    desired_ax = longitudinal_speed_pi_controller_parking_m(ego_status, parking_mission_info);
end

== matlab function generic_IVS/CarMaker/Subsystem/Final Project/Scenario 1/Subsystem9/Longiutidnal Control/Longitudinal PI Controller ==
  settings: updateMethod=DISCRETE  sampleTime=0.05
  data: desired_ax output; ego_status input Bus: busEgoVehicle; driving_mission_info input Bus: busDrivingMissionInfo
function desired_ax = longitudinal_speed_pi_controller_driving(ego_status, driving_mission_info)
    desired_ax = longitudinal_speed_pi_controller_driving_m(ego_status, driving_mission_info);
end

== matlab function generic_IVS/CarMaker/Subsystem/Final Project/Scenario 1/Subsystem8/MATLAB Function4 ==
  settings: sampleTime=0.1
  data: MapData_Info input Bus: busMapData; current_lane_info_in input Bus: busCurrentLaneInfo; current_lane_info_out output Bus: busCurrentLaneInfo; ego_status input Bus: busEgoVehicle
function current_lane_info_out  = current_lane_identifier(MapData_Info, current_lane_info_in, ego_status)
    current_lane_info_out  = current_lane_identifier_m(MapData_Info, current_lane_info_in, ego_status);
end

== matlab function generic_IVS/CarMaker/Subsystem/Final Project/Scenario 1/Subsystem8/Global Waypoints To Local Transfomer ==
  settings: sampleTime=0.05
  data: waypointList input; current_lane_info input Bus: busCurrentLaneInfo; local_waypoints_ output size=[30 2]; ego_status input Bus: busEgoVehicle
function local_waypoints_ = global_to_local_waypoints(waypointList, current_lane_info, ego_status)
    local_waypoints_ = global_to_local_waypoints_m(waypointList, current_lane_info, ego_status);
end

== matlab function generic_IVS/CarMaker/Subsystem/Final Project/Scenario 1/Subsystem8/MATLAB Function5 ==
  settings: sampleTime=0.001
  data: current_lane_info_out output Bus: busCurrentLaneInfo; current_lane_info_in input Bus: busCurrentLaneInfo; ego_status input
function current_lane_info_out = compute_lateral_info(current_lane_info_in, ego_status)
    current_lane_info_out = compute_lateral_info_m(current_lane_info_in, ego_status);
end

== matlab function generic_IVS/CarMaker/Subsystem/Final Project/Scenario 1/Subsystem8/MATLAB Function6 ==
  settings: sampleTime=0.05
  data: local_waypoints input; current_lane_info_out output Bus: busCurrentLaneInfo; current_lane_info_in input Bus: busCurrentLaneInfo
function current_lane_info_out = fit_polynomial_to_waypoints(local_waypoints, current_lane_info_in)
    current_lane_info_out = fit_polynomial_to_waypoints_m(local_waypoints, current_lane_info_in);
end

== matlab function generic_IVS/CarMaker/Subsystem/Final Project/Scenario 1/Subsystem9/Lateral Control/MATLAB Function7 ==
  settings: updateMethod=DISCRETE  sampleTime=0.05
  data: current_lane_info input Bus: busCurrentLaneInfo; ego_status input Bus: busEgoVehicle; delta output
function delta  = lateral_stanley_controller_(current_lane_info, ego_status)
    
    k_h = 0.8;
    k_e = 0.4;

    heading_error = atan(current_lane_info.lane_Coeff(2));
    cross_track_error = current_lane_info.y_lookAheadDistance;
    V = ego_status.ego_Speed;
    
    heading_err_term     = k_h * heading_error;
    cross_track_err_term = atan(k_e * cross_track_error / V);

    delta = (heading_err_term + cross_track_err_term);
    
    V_thresh = 1;
    if abs(V) < V_thresh
        delta = 0;
        return;
    end

end

== matlab function generic_IVS/CarMaker/Subsystem/Final Project/Scenario 1/Subsystem9/Lateral Control/MATLAB Function8 ==
  settings: updateMethod=DISCRETE  sampleTime=0.05
  data: current_lane_info input Bus: busCurrentLaneInfo; delta output
function delta  = lateral_PP_controller_driving(current_lane_info)
    delta  = lateral_PP_controller_driving_m(current_lane_info);
end
